simulink model "q6_TDO"  (R2020b)
settings: Solver=ode4  StartTime=0.0  StopTime=SIM_TIME  FixedStep=STEP_SIZE  RelTol=1e-3
undefined symbols (not defined in the file): F_tf_d, h, M, sigma_meas
libraries: cstblocks x8
settings Model: Creator=Theis  LastModifiedBy=Theis

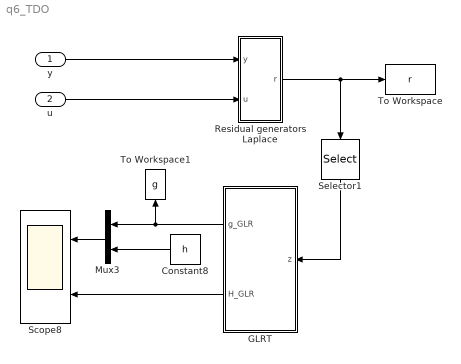
== system q6_TDO ==
  y : Inport
  u : Inport  Port=2
  Constant8 : Constant  Value=h
  GLRT : Subsystem
  Mux3 : Mux  Inputs=2
  Residual generators Laplace : Subsystem
  Scope8 : Scope  NumInputPorts=2
  Selector1 : Selector  InputPortWidth=4  IndexOptions=Index vector (dialog)  Indices=[2]  OutputSizes=1
  To Workspace : ToWorkspace  VariableName=r  SaveFormat=Timeseries  SampleTime=-1
  To Workspace1 : ToWorkspace  VariableName=g  SaveFormat=Timeseries  SampleTime=-1
  wires:
  Mux3/1 -> Scope8/1
  Residual generators Laplace/1(r) -> Selector1/1, To Workspace/1
  GLRT/1(g_GLR) -> Mux3/1, To Workspace1/1
  Selector1/1 -> GLRT/1(z)
  Constant8/1 -> Mux3/2
  GLRT/2(H_GLR) -> Scope8/2
  y/1 -> Residual generators Laplace/1(y)
  u/1 -> Residual generators Laplace/2(u)

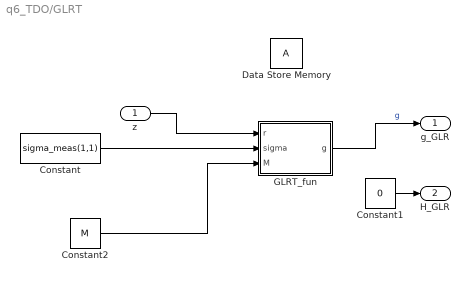
== system q6_TDO/GLRT ==
  z : Inport  OutDataTypeStr=double  PortDimensions=1
  Constant : Constant  Value=sigma_meas(1,1)
  Constant1 : Constant  Value=0
  Constant2 : Constant  Value=M
  Data Store Memory : DataStoreMemory  InitialValue=25  ShowAdditionalParam=off  OutDataTypeStr=double
  GLRT_fun : MATLAB Function  TreatAsAtomicUnit=on
  g_GLR : Outport  VectorParamsAs1DForOutWhenUnconnected=off
  H_GLR : Outport  Port=2  VectorParamsAs1DForOutWhenUnconnected=off
  wires:
  GLRT_fun/1(g) -> g_GLR/1  "g"
  z/1 -> GLRT_fun/1(r)
  Constant/1 -> GLRT_fun/2(sigma)
  Constant2/1 -> GLRT_fun/3(M)
  Constant1/1 -> H_GLR/1

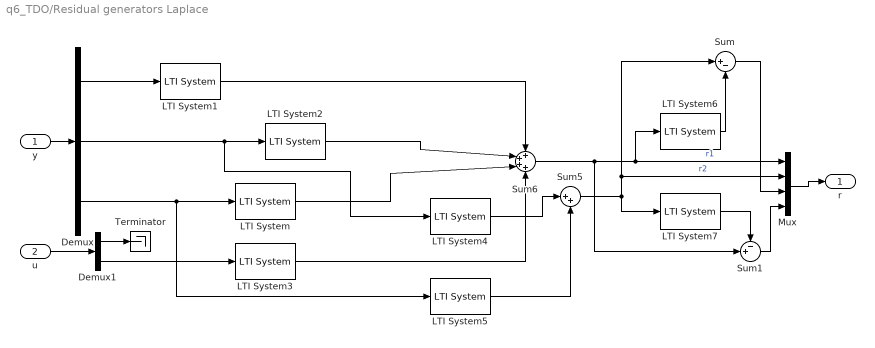
== system q6_TDO/Residual generators Laplace ==
  y : Inport  PortDimensions=3
  u : Inport  Port=2
  Demux : Demux  Outputs=3
  Demux1 : Demux  Outputs=2
  LTI System : cstblocks/LTI System  sys=F_tf_d(1,3)  IC=[]
  LTI System1 : cstblocks/LTI System  sys=F_tf_d(1,1)  IC=[]
  LTI System2 : cstblocks/LTI System  sys=F_tf_d(1,2)  IC=[]
  LTI System3 : cstblocks/LTI System  sys=F_tf_d(1,5)  IC=[]
  LTI System4 : cstblocks/LTI System  sys=F_tf_d(2,2)  IC=[]
  LTI System5 : cstblocks/LTI System  sys=F_tf_d(2,3)  IC=[]
  LTI System6 : cstblocks/LTI System  sys=r3_tf_d  IC=[]
  LTI System7 : cstblocks/LTI System  sys=r4_tf_d  IC=[]
  Mux : Mux
  Sum : Sum  Inputs=|+-
  Sum1 : Sum  Inputs=-+|
  Sum5 : Sum  Inputs=|++
  Sum6 : Sum  Inputs=++++
  Terminator : Terminator
  r : Outport  VectorParamsAs1DForOutWhenUnconnected=off
  wires:
  y/1 -> Demux/1
  Mux/1 -> r/1
  u/1 -> Demux1/1
  Demux1/1 -> Terminator/1
  Sum6/1 -> Sum1/2, LTI System6/1, Mux/1  "r1"
  Demux/1 -> LTI System1/1
  LTI System1/1 -> Sum6/1
  Demux/2 -> LTI System4/1, LTI System2/1
  LTI System2/1 -> Sum6/2
  Demux/3 -> LTI System5/1, LTI System/1
  LTI System/1 -> Sum6/3
  Demux1/2 -> LTI System3/1
  LTI System3/1 -> Sum6/4
  Sum5/1 -> Sum/1, Mux/2, LTI System7/1  "r2"
  LTI System4/1 -> Sum5/1
  LTI System5/1 -> Sum5/2
  LTI System6/1 -> Sum/2
  Sum/1 -> Mux/3
  Sum1/1 -> Mux/4
  LTI System7/1 -> Sum1/1

== matlab function q6_TDO/GLRT/GLRT_fun ==
  data: g output; A data_store_memory; r input; sigma input; M input
function g = glrt(r, sigma, M)
%#codegen

% global A

persistent Z;
persistent itr;

if isempty(itr)
    itr = 1;
end

if isempty(Z)
    Z = 0;
end

% Save latest residual value
Z = [Z; r];

n = length(Z);

% Decision function
mu0 = 0;


vec = zeros(1,M);
m = 0;
for j = (n-M+1):n
    m = m + 1;
    if j<1
        continue
    end

    runsum = 0;
    for i = j:n
        runsum = runsum + (Z(i)-mu0);
    end
    vec(m) = 1/(n - j + 1) * runsum.^2; 
end

g = 1/(2*sigma^2) * max(vec);


% maxSoFar = 0;
% 
% for i = 1:M
%     if n-i < 0
%         continue
%     end
%     
%     tmp = 1/i * sum( Z(n-i+1 : end) - mu0)^2;
%     if tmp > maxSoFar
%         maxSoFar = tmp;
%     end
% end
% 
% g = 1/(2*sigma^2) * maxSoFar;

% if itr == 10
%     disp(Z)
%     disp("----")
%     disp(r)
% end
% 
% itr = itr + 1;
